simulink model "flightControlSystem"  (R2022b)
settings: Solver=ode3  StartTime=0  StopTime=TFinal  FixedStep=Ts  RelTol=1e-3  EnableMultiTasking=on
undefined symbols (not defined in the file): codertarget, Controller, DiscIntNeverNeededParam, Discrete, Estimator, g, gray, init, orient_ref, pos_ref, Sensors, Time, Ts, var_acc_angle_N, var_bias_gyr_N, var_gyro_p_N, Vehicle
libraries: simulink x41, visiontextngfix x7, slpidlib x4, ctrlSharedLib x4, sharedtransform x3, visionanalysis x2, parrotlib x1
(part 3 of 3)

== system flightControlSystem/Control System/State Estimator/XY Position Estimator/EstimatorVelocity/AccelerationHandling ==
  dxy_estimin : Inport
  sensorIMU_datin : Inport  Port=2
  orient_estimin : Inport  Port=3
  Z_estimin : Inport  Port=4
  Add : Sum  Inputs=-+
  Bus Selector1 : BusSelector  OutputSignals=ddx,ddy,ddz
  Deactivate Acceleration If OF is not used due to low altitude : simulink/Logic and Bit Operations/Compare To Constant  relop=<=  const=Estimator.pos.opticalFlowZMax  OutDataTypeStr=boolean
  Logical Operator : Logic  Operator=OR  AllPortsSameDT=off  OutDataTypeStr=boolean
  Mux6 : Mux  Inputs=3
  Product : Product  Inputs=3
  Product1 : Product  Multiplication=Matrix(*)
  Rotation Angles to Direction Cosine Matrix : sharedtransform/Rotation Angles to Direction Cosine Matrix  rotationOrder=ZYX  aMode=aMode
  SelectPlanarddxy : Selector  InputPortWidth=3  IndexOptions=Index vector (dialog)  Indices=[1 2]  OutputSizes=1
  Selector : Selector  InputPortWidth=2  IndexOptions=Index vector (dialog)  Indices=1  OutputSizes=1
  Selector1 : Selector  InputPortWidth=2  IndexOptions=Index vector (dialog)  Indices=2  OutputSizes=1
  do not use acc if optical flow never available (Note OF@60Hz but ZOH to 200!) : simulink/Logic and Bit Operations/Compare To Constant  relop=~=  const=0  OutDataTypeStr=boolean
  do not use acc if optical flow never available (Note OF@60Hz but ZOH to 200!)1 : simulink/Logic and Bit Operations/Compare To Constant  relop=~=  const=0  OutDataTypeStr=boolean
  gainaccinput1 : Gain  OutDataTypeStr=single
  gravity : Constant  Value=[0 0 -g]
  acceleration_world : Outport  OutDataTypeStr=single  VectorParamsAs1DForOutWhenUnconnected=off
  wires:
  do not use acc if optical flow never available (Note OF@60Hz but ZOH to 200!)1/1 -> Logical Operator/2
  do not use acc if optical flow never available (Note OF@60Hz but ZOH to 200!)/1 -> Logical Operator/1
  Logical Operator/1 -> Product/1
  Selector1/1 -> do not use acc if optical flow never available (Note OF@60Hz but ZOH to 200!)1/1
  Selector/1 -> do not use acc if optical flow never available (Note OF@60Hz but ZOH to 200!)/1
  dxy_estimin/1 -> Selector1/1, Selector/1
  Product/1 -> acceleration_world/1
  Deactivate Acceleration If OF is not used due to low altitude/1 -> Product/3
  Z_estimin/1 -> Deactivate Acceleration If OF is not used due to low altitude/1
  Add/1 -> SelectPlanarddxy/1
  Product1/1 -> Add/1
  gravity/1 -> Product1/2
  SelectPlanarddxy/1 -> gainaccinput1/1
  Bus Selector1/3 -> Mux6/3  "<ddz>"
  Bus Selector1/1 -> Mux6/1  "<ddx>"
  sensorIMU_datin/1 -> Bus Selector1/1
  Mux6/1 -> Add/2
  Bus Selector1/2 -> Mux6/2  "<ddy>"
  orient_estimin/1 -> Rotation Angles to Direction Cosine Matrix/1
  Rotation Angles to Direction Cosine Matrix/1 -> Product1/1
  gainaccinput1/1 -> Product/2

== system flightControlSystem/Control System/State Estimator/XY Position Estimator/EstimatorVelocity/Angular velocity compensation for optical flow ==
  note: Optical flow readings are affected by both linear and angular velocity of the drone. We need to subtract the effect of angular velocity before using the flow data
  z_estimate : Inport
  Angular velocity w/o bias : Inport  Port=2
  Abs : Abs  SaturateOnIntegerOverflow=off
  Data Type Conversion : DataTypeConversion  SaturateOnIntegerOverflow=off  RndMeth=Floor
  Demux : Demux  Outputs=2
  Gain1 : Gain  Gain=-1
  Mux : Mux  Inputs=2
  Selector : Selector  InputPortWidth=3  IndexOptions=Index vector (dialog)  Indices=[1 2]  OutputSizes=1
  prod : Product  Inputs=**
  angular velocity correction : Outport
  wires:
  Gain1/1 -> Mux/1
  Mux/1 -> Data Type Conversion/1
  Demux/2 -> Gain1/1
  Data Type Conversion/1 -> angular velocity correction/1
  prod/1 -> Demux/1
  z_estimate/1 -> Abs/1
  Demux/1 -> Mux/2
  Selector/1 -> prod/2
  Abs/1 -> prod/1
  Angular velocity w/o bias/1 -> Selector/1

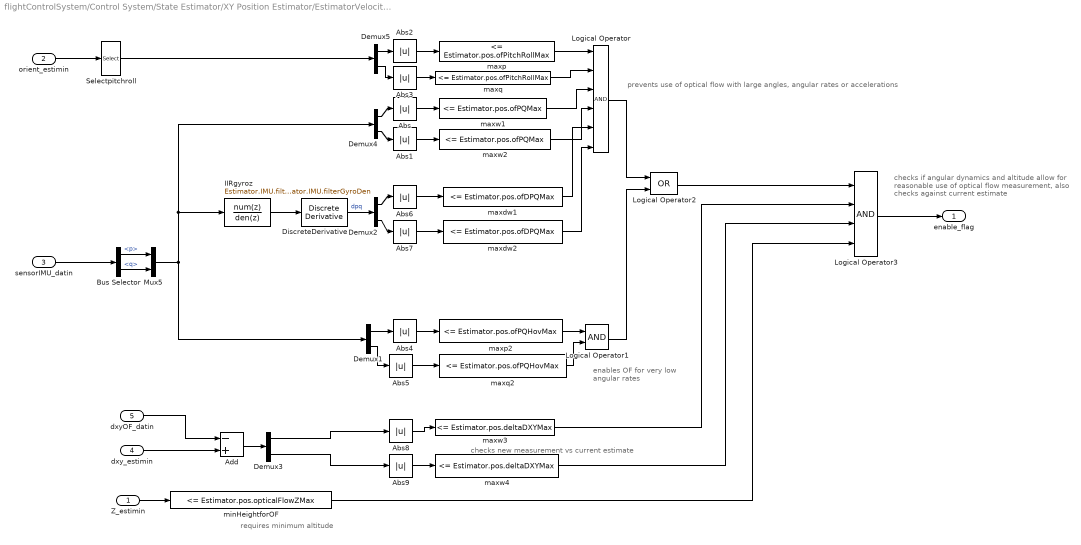
== system flightControlSystem/Control System/State Estimator/XY Position Estimator/EstimatorVelocity/DataHandling ==
  note: prevents use of optical flow with large angles, angular rates or accelerations
  note: enables OF for very
      | low angular rates
  note: checks if angular dynamics and altitude allow for
      | reasonable use of optical flow measurement,
      | also checks against current estimate
  note: checks new measurement vs current estimate
  note: requires minimum altitude
  Z_estimin : Inport
  orient_estimin : Inport  Port=2
  sensorIMU_datin : Inport  Port=3
  dxy_estimin : Inport  Port=4
  dxyOF_datin : Inport  Port=5
  Abs{,1..9} (10 alike) : Abs  SaturateOnIntegerOverflow=off
  Add : Sum  Inputs=-+
  Bus Selector : BusSelector  OutputSignals=p,q
  Demux{1..5} (5 alike) : Demux  Outputs=2
  DiscreteDerivative : simulink/Discrete/Discrete Derivative  gainval=1.0  ICPrevScaledInput=0.0  OutMin=[]  OutMax=[]  OutDataType=fixdt(1, 16)  OutScaling=2^-10  DoSatur=off
  IIRgyroz : DiscreteFilter  Numerator=Estimator.IMU.filterGyroNum  Denominator=Estimator.IMU.filterGyroDen
  Logical Operator : Logic  Inputs=6  AllPortsSameDT=off  OutDataTypeStr=boolean
  Logical Operator1 : Logic  AllPortsSameDT=off  OutDataTypeStr=boolean
  Logical Operator2 : Logic  Operator=OR  AllPortsSameDT=off  OutDataTypeStr=boolean
  Logical Operator3 : Logic  Inputs=4  AllPortsSameDT=off  OutDataTypeStr=boolean
  Mux5 : Mux  Inputs=2
  Selectpitchroll : Selector  InputPortWidth=3  IndexOptions=Index vector (dialog)  Indices=[2 3]  OutputSizes=1
  maxdw1 : simulink/Logic and Bit Operations/Compare To Constant  relop=<=  const=Estimator.pos.ofDPQMax  OutDataTypeStr=boolean
  maxdw2 : simulink/Logic and Bit Operations/Compare To Constant  relop=<=  const=Estimator.pos.ofDPQMax  OutDataTypeStr=boolean
  maxp : simulink/Logic and Bit Operations/Compare To Constant  relop=<=  const=Estimator.pos.ofPitchRollMax  OutDataTypeStr=boolean
  maxp2 : simulink/Logic and Bit Operations/Compare To Constant  relop=<=  const=Estimator.pos.ofPQHovMax  OutDataTypeStr=boolean
  maxq : simulink/Logic and Bit Operations/Compare To Constant  relop=<=  const=Estimator.pos.ofPitchRollMax  OutDataTypeStr=boolean
  maxq2 : simulink/Logic and Bit Operations/Compare To Constant  relop=<=  const=Estimator.pos.ofPQHovMax  OutDataTypeStr=boolean
  maxw1 : simulink/Logic and Bit Operations/Compare To Constant  relop=<=  const=Estimator.pos.ofPQMax  OutDataTypeStr=boolean
  maxw2 : simulink/Logic and Bit Operations/Compare To Constant  relop=<=  const=Estimator.pos.ofPQMax  OutDataTypeStr=boolean
  maxw3 : simulink/Logic and Bit Operations/Compare To Constant  relop=<=  const=Estimator.pos.deltaDXYMax  OutDataTypeStr=boolean
  maxw4 : simulink/Logic and Bit Operations/Compare To Constant  relop=<=  const=Estimator.pos.deltaDXYMax  OutDataTypeStr=boolean
  minHeightforOF : simulink/Logic and Bit Operations/Compare To Constant  relop=<=  const=Estimator.pos.opticalFlowZMax  OutDataTypeStr=boolean
  enable_flag : Outport  VectorParamsAs1DForOutWhenUnconnected=off
  wires:
  minHeightforOF/1 -> Logical Operator3/4
  IIRgyroz/1 -> DiscreteDerivative/1
  Mux5/1 -> Demux1/1, Demux4/1, IIRgyroz/1
  maxw4/1 -> Logical Operator3/3
  maxw3/1 -> Logical Operator3/2
  dxyOF_datin/1 -> Add/1
  Demux3/2 -> Abs9/1
  Demux3/1 -> Abs8/1
  dxy_estimin/1 -> Add/2
  Add/1 -> Demux3/1
  Abs9/1 -> maxw4/1
  Abs8/1 -> maxw3/1
  Logical Operator2/1 -> Logical Operator3/1
  Logical Operator3/1 -> enable_flag/1
  DiscreteDerivative/1 -> Demux2/1  "dpq"
  Demux2/2 -> Abs7/1
  Demux2/1 -> Abs6/1
  Abs7/1 -> maxdw2/1
  Abs6/1 -> maxdw1/1
  Logical Operator1/1 -> Logical Operator2/2
  Demux1/2 -> Abs5/1
  Demux1/1 -> Abs4/1
  Abs5/1 -> maxq2/1
  Abs4/1 -> maxp2/1
  Abs3/1 -> maxq/1
  Abs2/1 -> maxp/1
  Demux4/2 -> Abs1/1
  Demux4/1 -> Abs/1
  Abs1/1 -> maxw2/1
  Abs/1 -> maxw1/1
  Z_estimin/1 -> minHeightforOF/1
  Logical Operator/1 -> Logical Operator2/1
  maxw1/1 -> Logical Operator/3
  Bus Selector/1 -> Mux5/1  "<p>"
  Selectpitchroll/1 -> Demux5/1
  sensorIMU_datin/1 -> Bus Selector/1
  maxq2/1 -> Logical Operator1/2
  Bus Selector/2 -> Mux5/2  "<q>"
  maxp/1 -> Logical Operator/1
  maxw2/1 -> Logical Operator/4
  orient_estimin/1 -> Selectpitchroll/1
  maxdw1/1 -> Logical Operator/5
  maxdw2/1 -> Logical Operator/6
  maxq/1 -> Logical Operator/2
  Demux5/1 -> Abs2/1
  Demux5/2 -> Abs3/1
  maxp2/1 -> Logical Operator1/1

== system flightControlSystem/Control System/State Estimator/XY Position Estimator/EstimatorVelocity/xy velocity w//o angular velocity compensation ==
  note: Optical flow raw readings are converted to velocity in m/s based on the estimated altitude
  optical_flow : Inport
  z_estimate : Inport  Port=2
  " " : Product  Inputs=**
  Compare To Constant : simulink/Logic and Bit Operations/Compare To Constant  relop=<  const=200*4  OutDataTypeStr=boolean
  Counter Free-Running : simulink/Sources/Counter Free-Running  NumBits=32  tsamp=-1
  Gain : Gain  Gain=-1
  Select dxy : Selector  InputPortWidth=3  IndexOptions=Index vector (dialog)  Indices=[1 2]  OutputSizes=1
  Switch : Switch  Criteria=u2 > Threshold  SaturateOnIntegerOverflow=off  InputSameDT=off
  opticalFlowErrorCorrect : Gain  Gain=1.15
  optical_flow_dx_dy : Outport
  wires:
  Select dxy/1 -> optical_flow_dx_dy/1  "optical_flow_dx_dy"
  " "/1 -> opticalFlowErrorCorrect/1
  opticalFlowErrorCorrect/1 -> Switch/3
  Gain/1 -> " "/2
  Switch/1 -> Select dxy/1
  Counter Free-Running/1 -> Compare To Constant/1
  Compare To Constant/1 -> Switch/2
  optical_flow/1 -> " "/1, Switch/1
  z_estimate/1 -> Gain/1

== matlab function flightControlSystem/Control System/Path Planning/isCircleAligned ==
  data: direction input; land output; flag input; decision input; decicionCount input
function land = fcn(direction, flag, decision, decicionCount)
persistent landNow
if(isempty(landNow))
    landNow = false;
end
persistent landCount
if(isempty(landCount))
    landCount = 0;
end

center = [60,80];
distence = sqrt((center(1) - direction(1))^2 + (center(2) - direction(2))^2);

% 착륙 결심하면 무조건 착륙
if(landNow == true)
    land = true;
    return
end

% 원이 검출되면 착륙지점 거리 출력 
if(flag)
    fprintf("LANDING: DIST = %f\n", distence);
end

% 원이 검출됬고 거리가 특정값 이하이면 착륙 결정 카운트 + 1
if( distence < decision && flag)
    landCount = landCount + 1;

    % 이때 착륙 결정 카운트가 10보다 크면 착륙
    if(landCount > decicionCount)
        landNow = true;
    end
else

    % 거리가 특정값 보다 크면 착륙 카운트 -1
    landCount = landCount - 1;
end
if(landCount < 0)
    landCount = 0;
end

land = landNow;

== matlab function flightControlSystem/Control System/Path Planning/Control Output/MATLAB Function1 ==
  data: xin input; xout output; yin input; yout output; land input
function [xout,yout] = fcn(xin,yin,land)
if(land == true)
    xout = 0;
    yout = 0;
else
    xout = xin;
    yout = yin;
end

== matlab function flightControlSystem/Image Processing System/Subsystem/Circle Hough Transform ==
  data: direction output; u input; sensitivity input; Flag output; circle_max_value output; radius_threshold output
function [direction,Flag, circle_max_value,radius_threshold]  = fcn(u,sensitivity)
persistent flag;
if(isempty(flag))
    flag = 0;
end

accumulator = zeros(120,160);
theta = linspace(0,2*pi,100);
radii = 17.5;
radio = 30;
rows = 120;
columns = 160;
direction = [0,0];

for radi_range = radii:radio
    for row = 1: rows
        for col = 1: columns
            if(u(row,col) == 1)
                circle_col = int16(radi_range*cos(theta)+col);
                circle_row = int16(radi_range*sin(theta)+row);
                for k = 1:length(circle_col)
                    if (circle_col(k) > 0 && circle_row(k) > 0 && circle_col(k) <= columns && circle_row(k) <= rows)
                        accumulator(circle_row(k),circle_col(k)) = accumulator(circle_row(k),circle_col(k)) + 1;
                    end
                end
            end
        end
    end

    circle_max_value = max(accumulator,[],'all');
    radius_threshold = round(radi_range*2*pi*sensitivity);
    if (circle_max_value >= radius_threshold)
        [circle_center_row, circle_center_col] = find(accumulator == circle_max_value);
%         if(circle_center_row(1) < 60 && circle_center_col(1) > 70 && circle_center_col(1) < 90)
        flag = 1;
        direction(1,1) = circle_center_row(1);
        direction(1,2) = circle_center_col(1);
        break;
    end
    accumulator = zeros(120,160);
end
Flag = flag;

== matlab function flightControlSystem/Image Processing System/Landing Algorithm1/Circle Hough Transform ==
  data: accumulator output; u input; acc_max output; threshold input
function [accumulator,acc_max] = fcn(u,threshold)

radii = 17.5;
accumulator = zeros(120,160);
theta = linspace(0,2*pi,100);



for row = 1:120
    for col = 1:160
        if(u(row,col) > 0) % 선이 있는 좌표라면
            % 해당 픽셀을 중심으로 반지름이 radii 인원을 그린다.
            miniCircleX = radii*cos(theta)+col;
            miniCircleY = radii*sin(theta)+row;
            miniCircleX = int16(miniCircleX);
            miniCircleY = int16(miniCircleY);

            for idx = 1:length(miniCircleX)
                % 앞에서 그린 원이 인덱스 내부에 있다면
                if(miniCircleX(idx) >= 1 && miniCircleY(idx) >= 1 && miniCircleX(idx) <= 160 && miniCircleY(idx) <= 120)
                    accumulator(miniCircleY(idx),miniCircleX(idx)) = accumulator(miniCircleY(idx),miniCircleX(idx)) + 1;
                end
            end
        end
    end
end
acc_max = max(accumulator,[],"all");
%accumulator = accumulator ./ acc_max(1);
accumulator = accumulator ./ threshold;

== matlab function flightControlSystem/Image Processing System/Landing Algorithm ==
  data: u input; direction output; Flag output
function [direction, Flag] = fcn(u)
persistent circle_f;
persistent land;
persistent circle_direction;
if (isempty(land))
    land = 0;
end
if (isempty(circle_f))
    circle_f = 0;
end
if (isempty(circle_direction))
    circle_direction = [0,0];
end

radii = 15;
radio = 30;
sensitivity = 0.8;
theta = linspace(0,2*pi,100);
circle_find_mat = zeros(120,160);
rows = 120;
columns = 160;
if (land == 0)
    for radi_range = radii:radio
        radius_threshold = round(radi_range*2*pi*sensitivity);
        for row = 1: rows
            for col = 1: columns
                if(u(row,col) == 1)
                    circle_col = int16(radi_range*cos(theta)+col);
                    circle_row = int16(radi_range*sin(theta)+row);
                    for k = 1:length(circle_col)
                        if (circle_col(k) > 0 && circle_row(k) > 0 && circle_col(k) <= columns && circle_row(k) <= rows)
                            circle_find_mat(circle_row(k),circle_col(k)) = circle_find_mat(circle_row(k),circle_col(k)) + 1;
                        end
                    end
                end
            end
        end
        circle_max_value = max(circle_find_mat,[],'all');
        if (circle_max_value >= radius_threshold)
            [circle_center_row, circle_center_col] = find(circle_find_mat == circle_max_value);
            if(circle_center_row(1) < 60 && circle_center_col(1) > 70 && circle_center_col(1) < 90)
                circle_f = 1;
            end
            circle_direction(1,1) = circle_center_row(1);
            circle_direction(1,2) = circle_center_col(1);
            break
        end
    end
end

Flag = circle_f;
direction = circle_direction;

== matlab function flightControlSystem/Image Processing System/Mode_Select_Function1 ==
  data: u input; center_mat output; heading_mat output; output_mode output; yaw_out output; yaw_out2 output; roll_out output; slow_straight output; pts_erase_past_line output; pts_local_area output; pts_roi_circle output; pts_head_rectangle output; pts_center_rectangle output; pts_middle_rectangle output
function [center_mat, heading_mat, output_mode, yaw_out,yaw_out2, roll_out, slow_straight, pts_erase_past_line, pts_local_area, pts_roi_circle,pts_head_rectangle,pts_center_rectangle, pts_middle_rectangle] = fcn(u)

persistent local_cond;
persistent local_array;
persistent add_yaw;
persistent program_start;
persistent str_yaw_cond;

if (isempty(str_yaw_cond))
    str_yaw_cond = 0;
end

if (isempty(program_start))
    program_start = 0;
end

if (isempty(add_yaw))
    add_yaw = 0;
end

if (isempty(local_cond))
    local_cond = 0;
end

if (isempty(local_array))
    local_array = ones(4,1,'uint8');
end

%% Image Uploading Create Binary Matrix
s = size(u);
rows = s(1,1);
columns = s(1,2);
find_yaw_mat = zeros(rows, columns);

%% Reset Value
center = [60 80];

%% Center Matrix 
FOV = 15;
center_mat = u(center(1)-FOV:center(1)+FOV, center(2)-FOV:center(2)+FOV);
center_size = size(center_mat);
center_rows = center_size(1,1);
center_cols = center_size(1,2);

%% Heading_Matrix
rowFOV = 2*FOV;

head_up = 1;
head_down = head_up+rowFOV;
head_left = center(2) - FOV;
head_right = center(2) + FOV;

heading_mat = u(head_up:head_down, head_left:head_right);
heading_size = size(heading_mat);
head_rows = heading_size(1,1);
head_cols = heading_size(1,2);
head_one_num = nnz(heading_mat);
center_one_num = nnz(center_mat);

%% Middle Matrix
middle_up = head_down ;
middle_down = center(1) - FOV;
middle_left = head_left;
middle_right = head_right;
middle_mat = u(middle_up:middle_down, middle_left:middle_right);
middle_size = size(middle_mat);
middle_rows = middle_size(1,1);
middle_cols = middle_size(1,2);
middle_array = zeros(1,middle_rows);


count = 0;
for row = 1:middle_rows
    for col = 1:middle_cols
        if (middle_mat(row,col) == 1)
            count = count + 1;
            middle_array(1,count) = 1;
            break
        end
    end
end

middle_num = nnz(middle_array);

%% Slow Matrix
slow_up = 15;
slow_down = 45;
slow_left = middle_left;
slow_right = middle_right;
slow_mat = u(slow_up:slow_down, slow_left:slow_right);
slow_size = size(slow_mat);
slow_rows = slow_size(1,1);
slow_cols = slow_size(1,2);
slow_array = zeros(1,slow_rows);

count = 0;

for row = 1:slow_rows
    for col = 1:slow_cols
        if (slow_mat(row,col) == 1)
            count = count + 1;
            slow_array(1,count) = 1;
            break
        end
    end
end

slow_num = nnz(slow_array);

slow_straight = 0;
%% mode_Condition
heading_cond = (head_one_num > 0);

% True = Straingt_Mode, False = Yawing_Mode
center_cond = (center_one_num > 0);

%middle condition
middle_cond = (middle_num == middle_rows);

yaw_cond = ( heading_cond == 0 || (heading_cond == 1 && middle_cond == 0));

straight_cond = ( (heading_cond == 1 && middle_cond == 1) );
%% Mode_Selctor
yaw_out = 0;
output_mode = 0;
yaw_out2 = 0;
roll_out = 0;
r_min = 33; % circle_minimum_radius
r_max = 40; % circle_maximum_radius

del_height = 15;
del_width = 28;

del_left = round(center(2) - del_width/2);
del_right = del_left + del_width;
del_up = center(1) - del_height;

%% Straight Mode
if (straight_cond == 1 && center_cond == 1)
    local_cond = 0;
    local_array = ones(4,1, 'uint8');

    %% add_yaw Stop 및 실행 조건 생성

    left_side_top = 0;
    left_side_bottom = 0;
    right_side_top = 0;
    right_side_bottom = 0;

    for row = 1:head_rows
        for col = 1:head_cols
            if (heading_mat(row,col) == 1)
                if(col == 1)
                    break
                else
                    left_side_top = col;
                    break
                end
            end
        end
        if (not(left_side_top == 0))
            break
        end
    end        

    for row = head_rows:-1:1
        for col = 1:head_cols
            if (heading_mat(row,col) == 1)
                if(col == 1)
                    break
                else
                    left_side_bottom = col;
                    break
                end
            end
        end
        if (not(left_side_bottom == 0))
            break
        end
    end      

    for row = 1:head_rows
        for col = head_cols:-1:1
            if (heading_mat(row,col) == 1)
                if (col == head_cols)
                    break
                else
                    right_side_top = col;
                    break
                end
            end
        end
        if (not(right_side_top == 0))
            break
        end
    end

    for row = head_rows:-1:1
        for col = head_cols:-1:1
            if (heading_mat(row,col) == 1)
                if(col == head_cols)
                    break
                else
                    right_side_bottom = col;
                    break
                end
            end
        end
        if (not(right_side_bottom == 0))
            break
        end
    end
    no_right = (right_side_top == 0 && right_side_bottom == 0);
    no_left = (left_side_top == 0 && left_side_bottom == 0);
    yaw_FOV = 2;

    cw_yaw_left_stop = (left_side_bottom + yaw_FOV > left_side_top);
    cw_yaw_right_stop = (right_side_bottom + yaw_FOV > right_side_top);
    ccw_yaw_left_stop = (left_side_top + yaw_FOV > left_side_bottom);
    ccw_yaw_right_stop = (right_side_top + yaw_FOV > right_side_bottom);
    
    if(add_yaw == 1)
        if(no_right == 1)
            if(cw_yaw_left_stop == 1)
                add_yaw = 0;
            end
        elseif(no_left == 1)
            if(cw_yaw_right_stop == 1)
                add_yaw = 0;
            end
        else
            if(cw_yaw_left_stop == 1)
                add_yaw = 0;
            end
        end
        yaw_out2 = 1;

    elseif(add_yaw == -1)
        if(no_right == 1)
            if(ccw_yaw_left_stop == 1)
                add_yaw = 0;
            end
        elseif(no_left == 1)
            if(ccw_yaw_right_stop == 1)
                add_yaw = 0;
            end
        else
            if(ccw_yaw_right_stop == 1)
                add_yaw = 0;
            end
        end
        yaw_out2 = -1;

        %% Straight Decision
    elseif(add_yaw == 0)

        % Center_yaw_cond , Roll_condition
        center_left_top = 0;
        center_left_bottom = 0;
        center_right_top = 0;
        center_right_bottom = 0;
        
        for row = 1:center_rows
            for col = 1:center_cols
                if (center_mat(row,col) == 1)
                    center_left_top = col;
                    break
                end
            end
            if (not(center_left_top == 0))
                break
            end
        end        

        for row = center_rows:-1:1
            for col = 1:center_cols
                if (center_mat(row,col) == 1)
                    center_left_bottom = col;
                    break
                end
            end
            if (not(center_left_bottom == 0))
                break
            end
        end      
        
        for row = 1:center_rows
            for col = center_cols:-1:1
                if (center_mat(row,col) == 1)
                    center_right_top = col;
                    break
                end
            end
            if (not(center_right_top == 0))
                break
            end
        end
        
        for row = center_rows:-1:1
            for col = center_cols:-1:1
                if (center_mat(row,col) == 1)
                    center_right_bottom = col;
                    break
                end
            end
            if (not(center_right_bottom == 0))
                break
            end
        end
        
        straight_yaw_FOV = 2;
        
        if(center_left_bottom == 1 && center_left_top == 1)
            center_right_cond = (center_right_bottom + straight_yaw_FOV < center_right_top);
            center_left_cond = (center_right_top + straight_yaw_FOV < center_right_bottom);
        elseif(center_right_bottom == center_cols && center_right_top == center_cols)
            center_right_cond = (center_left_bottom + straight_yaw_FOV < center_left_top);
            center_left_cond = (center_left_top + straight_yaw_FOV < center_left_bottom); 
        else
            center_right_cond = (center_left_bottom + straight_yaw_FOV  < center_left_top);
            center_left_cond = (center_right_top + straight_yaw_FOV < center_right_bottom);
        end
        
        
        center_right_mean = (center_right_top + center_right_bottom)/2;
        center_left_mean = (center_left_top + center_left_bottom)/2;
        roll_FOV = 3; 
        
        % 계속 직진 판단
        only_straight_cond = ((center_right_top - center_left_top) > center_cols - round(2.5*roll_FOV)) || ((center_left_bottom - center_right_bottom) > center_cols - round(2.5*roll_FOV)); 
        

        if(no_left == 1)
            right_yaw_cond = (right_side_bottom + yaw_FOV < right_side_top);
            left_yaw_cond = (right_side_top + yaw_FOV < right_side_bottom);
        elseif (no_right == 1)
            right_yaw_cond = (left_side_bottom + yaw_FOV < left_side_top);
            left_yaw_cond = (left_side_top + yaw_FOV < left_side_bottom);
        else
            right_yaw_cond = (left_side_bottom + yaw_FOV < left_side_top);
            left_yaw_cond = (right_side_top + yaw_FOV < right_side_bottom);
        end

        %% Slow Straight Cond
        if(slow_num < slow_rows)
            slow_straight = 1;
        end

        %% Straight_Output Part
        if (right_yaw_cond && center_right_cond)
            add_yaw = 1;
        elseif (left_yaw_cond && center_left_cond)
            add_yaw = -1;
        else

            % Center Line Recover Using Rolling
            if (only_straight_cond == 0)
                if (center_right_mean > center_cols - roll_FOV)
                    roll_out = 1;
                    output_mode = 1;% Right_Moving
                elseif (center_left_mean < roll_FOV)
                    roll_out = -1;
                    output_mode = 1;% Left_moving
                else
                    output_mode = 1;
                end
                str_yaw_cond = 1;
            else
                output_mode = 1; % Straight_moving
                str_yaw_cond = 1;
                if(program_start == 0) % Drone이 이동하기 시작
                    program_start = 1;
                end
            end
        end
    end

%% Yawing_Mode
elseif (yaw_cond == 1 && center_cond == 1)

    direction_of_nextLine = 0;
    %% 요잉 지점 찾은 후부터 시작
    if (local_cond == 1)
        %% 국소 지점 imgage 생성
        row_min = local_array(1);
        row_max = local_array(2);
        col_min = local_array(3);
        col_max = local_array(4);
        find_yaw_mat(row_min:row_max, col_min:col_max) = u(row_min:row_max, col_min:col_max);

    end
    %% Main 이미지 프로세싱 부분
    local_area = ones(4,1,'uint8'); % (1) = row_min, (2) = row_max, (3) = col_min (4) = col_max
    count = 0;
    for row = 1:rows 
        for col = 1:columns    

            distance_from_center =  sqrt((row-center(1))^2 + (col - center(2))^2);
            is_past_line_area = (col > (del_left)) && (col < (del_right))  && (row > (del_up));

            if (local_cond == 0 && distance_from_center <= r_max && distance_from_center >= r_min) % First_Loop
                if (u(row,col) == 1 && not(is_past_line_area))
                    count = count + 1;

                    if (count == 1)  % 첫번째 탐색 때, 값 초기화
                        local_area(1) = row;
                        local_area(2) = row;
                        local_area(3) = col;
                        local_area(4) = col;
                    end

                    if (local_area(1) > row) % row_min
                        local_area(1) = row;
                    end

                    if (local_area(2) < row) % row_max
                        local_area(2) = row;
                    end

                    if (local_area(3) > col) % col_min
                        local_area(3) = col;
                    end

                    if (local_area(4) < col) % col_max
                        local_area(4) = col;
                    end
                end
         
            elseif (local_cond == 1 && distance_from_center <= r_max && distance_from_center >= r_min)  % Main_Loop
                if (find_yaw_mat(row,col) == 1)
                    count = count + 1;

                    if (count == 1)  % 첫번째 탐색 때, 값 초기화
                        local_area(1) = row;
                        local_area(2) = row;
                        local_area(3) = col;
                        local_area(4) = col;
                    end
                    
                    direction_of_nextLine = direction_of_nextLine + col;

                   if (row < local_area(1)) % row_min
                       local_area(1) = row;
                   end

                   if (row > local_area(2)) % row_max
                       local_area(2) = row;
                   end

                   if (col < local_area(3)) % col_min
                       local_area(3) = col;
                   end

                   if (col > local_area(4)) % col_max
                       local_area(4) = col;
                   end
                end
            end
        end
    end
    %% Start Line이 드론 뒤에 있을경우 Yaw 결정
    start_yaw_cond = 0;

    if (program_start == 0)
        if(local_area(1) == 1 && local_area(2) == 1 && local_area(3) == 1 && local_area(4) == 1)
            start_yaw_cond = 1;
        end
    end

    if (local_cond == 1) % Main_Loop_end
        direction_of_nextLine = direction_of_nextLine/count;
    end

    if (start_yaw_cond == 0)
        local_cond = 1;
    end

    %% local_array에 4 Point 할당
    local_FOV = 5;
    if (start_yaw_cond == 0)
        if (local_area(1) < local_FOV + 1)
            local_array(1) = local_area(1);
        else
            local_array(1) = local_area(1) - local_FOV;
        end
    
        if (local_area(2) > rows - local_FOV)
            local_array(2) = local_area(2);
        else
            local_array(2) = local_area(2) + local_FOV;
        end
    
        if (local_area(3) < local_FOV + 1)
            local_array(3) = local_area(3);
        else
            local_array(3) = local_area(3) - local_FOV;
        end
    
        if (local_area(4) > columns - local_FOV)
            local_array(4) = local_area(4);
        else
            local_array(4) = local_area(4) + local_FOV;
        end
    end

    %% yawing output 구간
    if (direction_of_nextLine == 0 && start_yaw_cond == 0)
        yaw_out = 0;
    elseif (direction_of_nextLine > center(2))
        yaw_out = 1; % Right = 1
        add_yaw = 1;
    elseif (direction_of_nextLine <= center(2))
        yaw_out = -1; % Left = -1\
        add_yaw=-1;
    end
    str_yaw_cond = 0;
else
    disp("EXCEPTION : Mode condition Exception")
end

%% 화면에 Draw Shape 를 이용해 이미지 처리 시각화

pts_erase_past_line = int32([del_left, del_up, del_width, columns - del_up]);
pts_roi_circle = int32([center(2),center(1),r_max; center(2),center(1),r_min]);
pts_head_rectangle = int32([head_left,head_up,head_right-head_left,head_down-head_up]);
pts_center_rectangle = int32([center(2)-FOV,center(1)-FOV, 2*FOV,2*FOV]);
pts_middle_rectangle = int32([middle_left,middle_up, middle_right - middle_left, middle_down - middle_up]);
if(length(local_array) == 4 && heading_cond == 0 && center_cond == 1 )
    pts_local_area = int32([local_array(3), local_array(1), local_array(4) - local_array(3), local_array(2) - local_array(1)]);
else
    pts_local_area = int32([0 0 0 0]);
end

%% Center Matrix = None .. 빨간색 라인 위에 없을때
if (center_cond == 0)
    row_mean = 0;
    col_mean = 0;
    count = 0;
    for row = 1:rows 
        for col = 1:columns
            if(u(row,col) == 1)
               count = count + 1;
               row_mean = row_mean + row;
               col_mean = col_mean + col;
            end
        end
    end
    row_mean = round(row_mean/count);
    col_mean = round(col_mean/count);
    if (row_mean < center(1) - 3)
        output_mode = 1;
    elseif (row_mean > center(1) + 3)
        output_mode = -1;
    elseif ( col_mean < center(2) - 3)
        roll_out = -2;
    elseif ( col_mean > center(2) + 3)
        roll_out = 2;
    end
    return
end

== matlab function flightControlSystem/Image Processing System/Landing Algorithm1/Threshold ==
  data: u input; BW output; threshold_gain input
function BW = fcn(u,threshold_gain)
BW = imbinarize(u,threshold_gain);

== matlab function flightControlSystem/Image Processing System/View Process/convert ==
  data: u input; y output
function y = fcn(u)

y=  int16([0 0]);
y(1) = u(2);
y(2) = u(1);

== matlab function flightControlSystem/Image Processing System/Landing Algorithm1/Circle Detect ==
  data: u input; land output; landingGain input; Flag output; direction output
function [land, Flag, direction ] = fcn(u,landingGain)

persistent detectCount
if(isempty(detectCount))
    detectCount = 0;
end
persistent flag
if(isempty(flag))
    flag = false;
end
persistent circle_location
if(isempty(circle_location))
    circle_location = [0 0];
end

persistent landNow
if(isempty(landNow))
    landNow = false;
end

%% 상수 선언
center = [60 80];
circleDetectedCount = 10;

%% 작동 부분 
if(landNow == true)
    land = landNow;
    direction = circle_location;
    Flag = flag;
    return;
end

if(nnz(u) > 0 && flag == false)
    detectCount = detectCount + 1;
    if(detectCount > circleDetectedCount)
        flag = true;
    end

elseif(nnz(u) > 0 && flag == true)
    pointIdx = [0 0]; % pointIdx(1) = row, pointIdx(2) = col
    
    % 원검출 이미지 영상에서 원의 중심으로 추정되는 픽셀의 위치 구하기
    count = 0;
    for row = 1:120
        for col = 1:160
            if(u(row,col) == 1)
                pointIdx(1) = pointIdx(1) + row;
                pointIdx(2) = pointIdx(2) + col;
                count = count + 1;
            end
        end
    end
    % 위에 것을 바탕으로 착륙 지점 구하기
    circle_location = [round(pointIdx(1)/count), round(pointIdx(2)/count)];
    
    % 착륙지점에 도착했는지
    distance_to_circle = sqrt(circle_location(1)^2 + circle_location(2)^2);
    if(distance_to_circle < landingGain) % landingGain은 착륙 조건의 민감도를 나타내고 클수록 부정확한 착륙
        landNow = true;
    else
        landNow = false;
    end
else % 착륙 조건 아님
    landNow = false;
    detectCount = 0;
    
end
land = landNow;
direction = circle_location;
Flag = flag;
%count = detectCount;

== matlab function flightControlSystem/Control System/Controller/Position Controller/Position error transformation (Earth to Body frame) ==
  data: yaw input; xy_err_earth input; xy_err_body output
function xy_err_body = fcn(yaw,xy_err_earth)

transformation = [cos(yaw), sin(yaw); -sin(yaw),  cos(yaw)];
xy_err_body = transformation * xy_err_earth;


end

== matlab function flightControlSystem/Control System/Path Planning/Flying Commend Generator/MATLAB Function ==
  data: yaw input; output_mode input; xout output; yout output; roll input; roll_value input; str_value input
function [xout, yout] = fcn(yaw, output_mode, roll, roll_value, str_value)
xout = 0;
yout = 0;

if (output_mode == 0)
    xout = 0 * cos(yaw);
    yout = 0 * sin(yaw);
elseif (output_mode == 1)
    if (roll == 0)
        xout = str_value * cos(yaw);
        yout = str_value * sin(yaw); 
    elseif (roll == 1)
        xout = str_value * cos(yaw)  + roll_value * cos(yaw + (pi/2));
        yout = str_value * sin(yaw)  + roll_value * sin(yaw + (pi/2));
    elseif (roll == -1)
        xout = str_value * cos(yaw)  - roll_value * cos(yaw + (pi/2));
        yout = str_value * sin(yaw)  - roll_value * sin(yaw + (pi/2)); 
    end
elseif ( output_mode == -1)
    xout = -1 * cos(yaw);
    yout = -1 * sin(yaw);
elseif ( output_mode == 3)
    xout = 0.5 * cos(yaw);
    yout = 0.5 * sin(yaw);
elseif ( output_mode == -3)
    xout = -0.5 * cos(yaw);
    yout = -0.5 * sin(yaw);
end

== matlab function flightControlSystem/Control System/Path Planning/Landing Command Generator/CalcTheta ==
  data: direct input; xout output; flag input; yout output; yaw input
function [xout, yout] = fcn(direct, flag, yaw)
center = [60 80];

if(flag && length(direct) == 2)
    dx = direct(1)-center(1);
    dy = direct(2)-center(2);
    xout = dx*cos(yaw);
    yout = dy*sin(yaw);
else
    xout = 0;
    yout = 0;
end

== matlab function flightControlSystem/Control System/Path Planning/Decent Rate Controller/Softlanding/Shutdown ==
  data: k input; z output
function z = fcn(k)
if(k > -0.7)
    z = 0
else
    z = k
end

== matlab function flightControlSystem/Image Processing System/Subsystem/Circle Detect ==
  data: detected input; Flag output
function Flag  = fcn(detected)

persistent detectCount
if(isempty(detectCount))
    detectCount = 0;
end
persistent flag
if(isempty(flag))
    flag = false;
end
persistent circle_location
if(isempty(circle_location))
    circle_location = [0 0];
end


%% 상수 선언
circleDetectedCount = 10;

%% 작동 부분 
if(flag == true)
    Flag = flag;
    return
end

if(detected > 0 && flag == false)
    detectCount = detectCount + 1;
    if(detectCount > circleDetectedCount)
        flag = true;
    end
    
else % 착륙 조건 아님
    detectCount = 0;
    flag = false;
end

Flag = flag;
%count = detectCount;
